simulink model "HPF"  (R2022a)
settings: Solver=VariableStepAuto  StartTime=0.0  StopTime=10.0  FixedStep=.000000001  RelTol=1e-3
values from neighbouring files (symbols this model uses):
  HPF_Sine_Amplitude = 1    [Run_Sim_HPF.m]
  HPF_Sine_Freq = 100    [Run_Sim_HPF.m]
  Vary_Sine_Feq = Start_Freq:step:End_Freq    [Run_Sim_HPF.m]
libraries: dspfdesign x7, dspsrcs4 x5
settings Model: Creator=chadw  LastModifiedBy=chadw

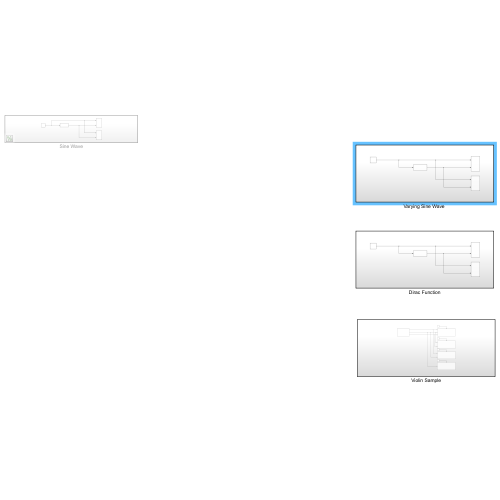
[thumbnail: Simulink's stored preview of the top-level diagram]
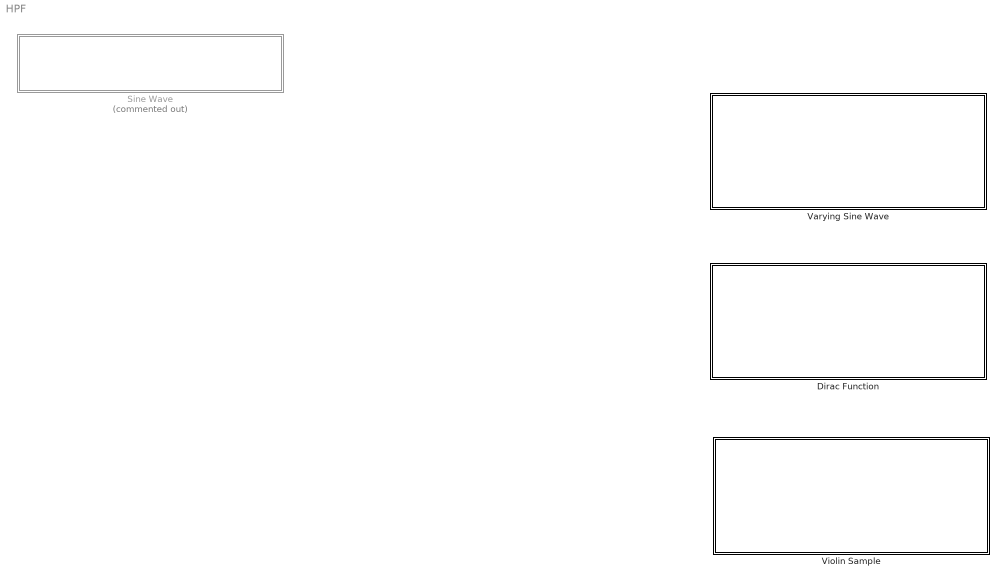
== system HPF ==
  Dirac Function : Subsystem
  Sine Wave : Subsystem  Commented=on
  "Varying Sine Wave " : Subsystem
  Violin Sample : Subsystem

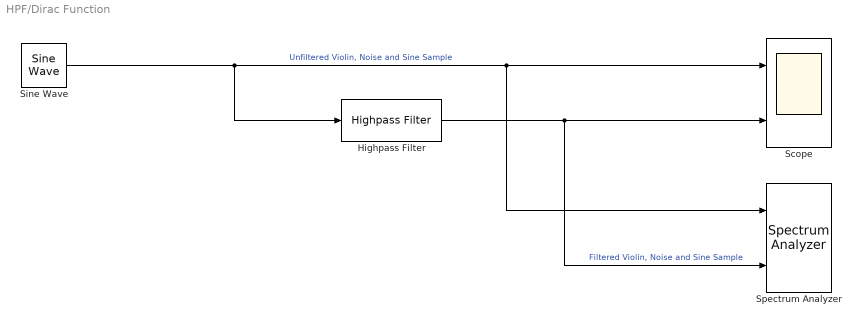
== system HPF/Dirac Function ==
  Highpass Filter : dspfdesign/Highpass Filter  FilterType=FIR  DesignForMinimumOrder=on  FilterOrder=50  StopbandFrequency=HPF_StopBand_Freq  PassbandFrequency=HPF_PassBand_Freq  StopbandAttenuation=HPF_StopBand_Amp  PassbandRipple=HPF_PassBand_Amp  InheritSampleRate=off  SampleRate=44100  SimulateUsing=Interpreted execution  roundingMode=Floor  coeffsDataTypeStr=fixdt(1,16)
  Scope : Scope  NumInputPorts=2
  Sine Wave : dspsrcs4/Sine Wave  Amplitude=1  Frequency=Vary_Sine_Feq  Phase=0  SampleMode=Discrete  OutComplex=Real  CompMethod=Trigonometric fcn  TableSize=Speed  SampleTime=1/1000  SamplesPerFrame=1  ResetState=Restart at time zero  OutputFrames=off  dataType=double  wordLen=16  udDataType=sfix(16)  fracBitsMode=Best precision  numFracBits=15  OutDataTypeStr=double  LastOutDataTypeStr=double
  Spectrum Analyzer : SpectrumAnalyzer  NumInputPorts=2
  wires:
  Sine Wave/1 -> Spectrum Analyzer/1, Scope/1, Highpass Filter/1  "Unfiltered Violin, Noise and Sine Sample"
  Highpass Filter/1 -> Spectrum Analyzer/2, Scope/2  "Filtered Violin, Noise and Sine Sample"

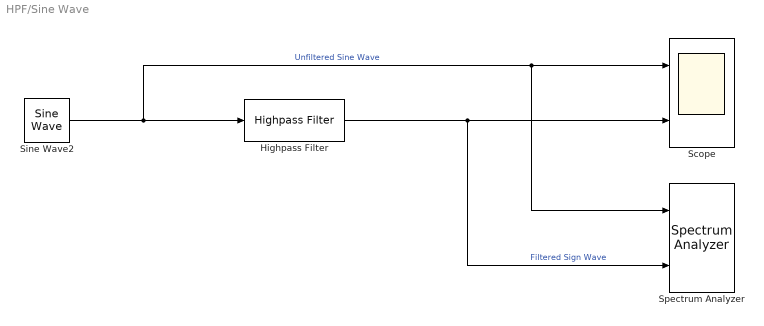
== system HPF/Sine Wave ==
  Highpass Filter : dspfdesign/Highpass Filter  FilterType=FIR  DesignForMinimumOrder=on  FilterOrder=50  StopbandFrequency=HPF_StopBand_Freq  PassbandFrequency=HPF_PassBand_Freq  StopbandAttenuation=HPF_StopBand_Amp  PassbandRipple=HPF_PassBand_Amp  InheritSampleRate=off  SampleRate=44100  SimulateUsing=Interpreted execution  roundingMode=Floor  coeffsDataTypeStr=fixdt(1,16)
  Scope : Scope  NumInputPorts=2
  Sine Wave2 : dspsrcs4/Sine Wave  Amplitude=HPF_Sine_Amplitude  Frequency=HPF_Sine_Freq  Phase=0  SampleMode=Discrete  OutComplex=Real  CompMethod=Trigonometric fcn  TableSize=Speed  SampleTime=1/1000  SamplesPerFrame=1  ResetState=Restart at time zero  OutputFrames=off  dataType=double  wordLen=16  udDataType=sfix(16)  fracBitsMode=Best precision  numFracBits=15  OutDataTypeStr=double  LastOutDataTypeStr=double
  Spectrum Analyzer : SpectrumAnalyzer  NumInputPorts=2
  wires:
  Sine Wave2/1 -> Scope/1, Spectrum Analyzer/1, Highpass Filter/1  "Unfiltered Sine Wave"
  Highpass Filter/1 -> Spectrum Analyzer/2, Scope/2  "Filtered Sign Wave"

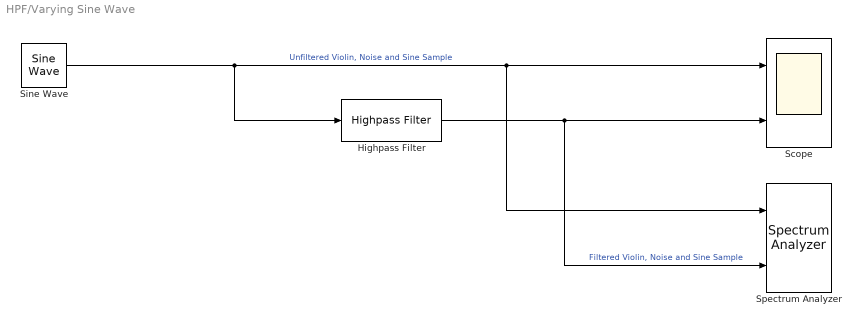
== system HPF/Varying Sine Wave  ==
  Highpass Filter : dspfdesign/Highpass Filter  FilterType=FIR  DesignForMinimumOrder=on  FilterOrder=50  StopbandFrequency=HPF_StopBand_Freq  PassbandFrequency=HPF_PassBand_Freq  StopbandAttenuation=HPF_StopBand_Amp  PassbandRipple=HPF_PassBand_Amp  InheritSampleRate=off  SampleRate=44100  SimulateUsing=Interpreted execution  roundingMode=Floor  coeffsDataTypeStr=fixdt(1,16)
  Scope : Scope  NumInputPorts=2
  Sine Wave : dspsrcs4/Sine Wave  Amplitude=1  Frequency=Vary_Sine_Feq  Phase=0  SampleMode=Discrete  OutComplex=Real  CompMethod=Trigonometric fcn  TableSize=Speed  SampleTime=1/1000  SamplesPerFrame=1  ResetState=Restart at time zero  OutputFrames=off  dataType=double  wordLen=16  udDataType=sfix(16)  fracBitsMode=Best precision  numFracBits=15  OutDataTypeStr=double  LastOutDataTypeStr=double
  Spectrum Analyzer : SpectrumAnalyzer  NumInputPorts=2
  wires:
  Highpass Filter/1 -> Scope/2, Spectrum Analyzer/2  "Filtered Violin, Noise and Sine Sample"
  Sine Wave/1 -> Highpass Filter/1, Scope/1, Spectrum Analyzer/1  "Unfiltered Violin, Noise and Sine Sample"

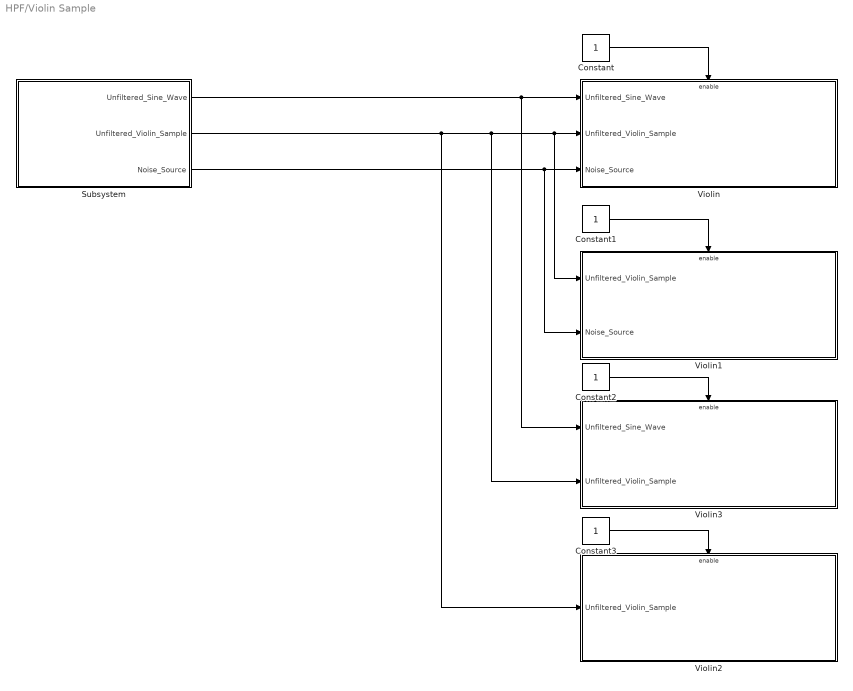
== system HPF/Violin Sample ==
  Constant{,1..3} (4 alike) : Constant  OutDataTypeStr=boolean
  Subsystem : Subsystem
  Violin : Subsystem
  Violin1 : Subsystem
  Violin2 : Subsystem
  Violin3 : Subsystem
  wires:
  Constant/1 -> Violin/Enable
  Subsystem/2(Unfiltered_Violin_Sample) -> Violin2/1(Unfiltered_Violin_Sample), Violin3/2(Unfiltered_Violin_Sample), Violin1/1(Unfiltered_Violin_Sample), Violin/2(Unfiltered_Violin_Sample)
  Constant3/1 -> Violin2/Enable
  Subsystem/1(Unfiltered_Sine_Wave) -> Violin3/1(Unfiltered_Sine_Wave), Violin/1(Unfiltered_Sine_Wave)
  Subsystem/3(Noise_Source) -> Violin1/2(Noise_Source), Violin/3(Noise_Source)
  Constant1/1 -> Violin1/Enable
  Constant2/1 -> Violin3/Enable

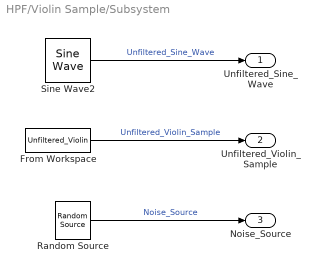
== system HPF/Violin Sample/Subsystem ==
  From Workspace : FromWorkspace  VariableName=Unfiltered_Violin  SampleTime=-1
  Random Source : dspsrcs4/Random Source  SrcType=Uniform  NormMethod=Ziggurat  CltLength=12  MinVal=0  MaxVal=1  MeanVal=0  VarVal=1  RepMode=Not repeatable  rawSeed=1  IsInherit=off  SampMode=Discrete  SampTime=1  SampFrame=1  DataType=Double  OutComplex=Real  OutputFrames=off
  Sine Wave2 : dspsrcs4/Sine Wave  Amplitude=HPF_Sine_Amplitude  Frequency=HPF_Sine_Freq  Phase=0  SampleMode=Discrete  OutComplex=Real  CompMethod=Trigonometric fcn  TableSize=Speed  SampleTime=1/1000  SamplesPerFrame=1  ResetState=Restart at time zero  OutputFrames=off  dataType=double  wordLen=16  udDataType=sfix(16)  fracBitsMode=Best precision  numFracBits=15  OutDataTypeStr=double  LastOutDataTypeStr=double
  Unfiltered_Sine_Wave : Outport
  Unfiltered_Violin_Sample : Outport  Port=2
  Noise_Source : Outport  Port=3
  wires:
  Random Source/1 -> Noise_Source/1  "Noise_Source"
  Sine Wave2/1 -> Unfiltered_Sine_Wave/1  "Unfiltered_Sine_Wave"
  From Workspace/1 -> Unfiltered_Violin_Sample/1  "Unfiltered_Violin_Sample"

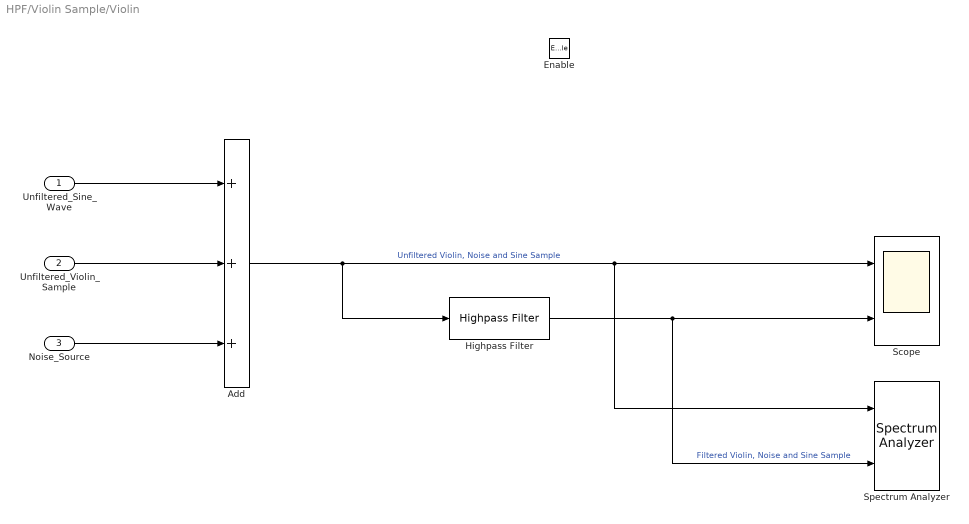
== system HPF/Violin Sample/Violin ==
  Unfiltered_Sine_Wave : Inport
  Unfiltered_Violin_Sample : Inport  Port=2
  Noise_Source : Inport  Port=3
  Enable : EnablePort
  Add : Sum  Inputs=3
  Highpass Filter : dspfdesign/Highpass Filter  FilterType=FIR  DesignForMinimumOrder=on  FilterOrder=50  StopbandFrequency=HPF_StopBand_Freq  PassbandFrequency=HPF_PassBand_Freq  StopbandAttenuation=HPF_StopBand_Amp  PassbandRipple=HPF_PassBand_Amp  InheritSampleRate=off  SampleRate=44100  SimulateUsing=Interpreted execution  roundingMode=Floor  coeffsDataTypeStr=fixdt(1,16)
  Scope : Scope  NumInputPorts=2
  Spectrum Analyzer : SpectrumAnalyzer  NumInputPorts=2
  wires:
  Highpass Filter/1 -> Scope/2, Spectrum Analyzer/2  "Filtered Violin, Noise and Sine Sample"
  Add/1 -> Highpass Filter/1, Scope/1, Spectrum Analyzer/1  "Unfiltered Violin, Noise and Sine Sample"
  Unfiltered_Sine_Wave/1 -> Add/1
  Unfiltered_Violin_Sample/1 -> Add/2
  Noise_Source/1 -> Add/3

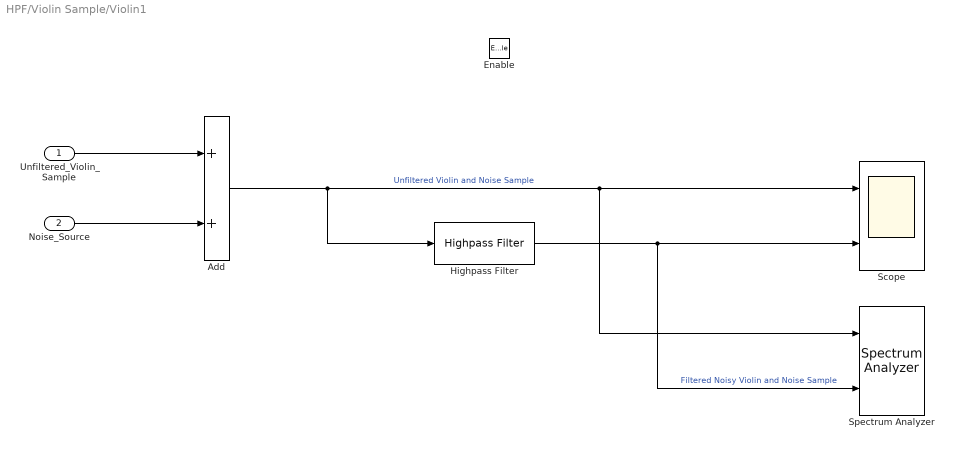
== system HPF/Violin Sample/Violin1 ==
  Unfiltered_Violin_Sample : Inport
  Noise_Source : Inport  Port=2
  Enable : EnablePort
  Add : Sum  Inputs=2
  Highpass Filter : dspfdesign/Highpass Filter  FilterType=FIR  DesignForMinimumOrder=on  FilterOrder=50  StopbandFrequency=HPF_StopBand_Freq  PassbandFrequency=HPF_PassBand_Freq  StopbandAttenuation=HPF_StopBand_Amp  PassbandRipple=HPF_PassBand_Amp  InheritSampleRate=off  SampleRate=44100  SimulateUsing=Interpreted execution  roundingMode=Floor  coeffsDataTypeStr=fixdt(1,16)
  Scope : Scope  NumInputPorts=2
  Spectrum Analyzer : SpectrumAnalyzer  NumInputPorts=2
  wires:
  Noise_Source/1 -> Add/2
  Add/1 -> Highpass Filter/1, Spectrum Analyzer/1, Scope/1  "Unfiltered Violin and Noise Sample"
  Highpass Filter/1 -> Spectrum Analyzer/2, Scope/2  "Filtered Noisy Violin and Noise Sample"
  Unfiltered_Violin_Sample/1 -> Add/1

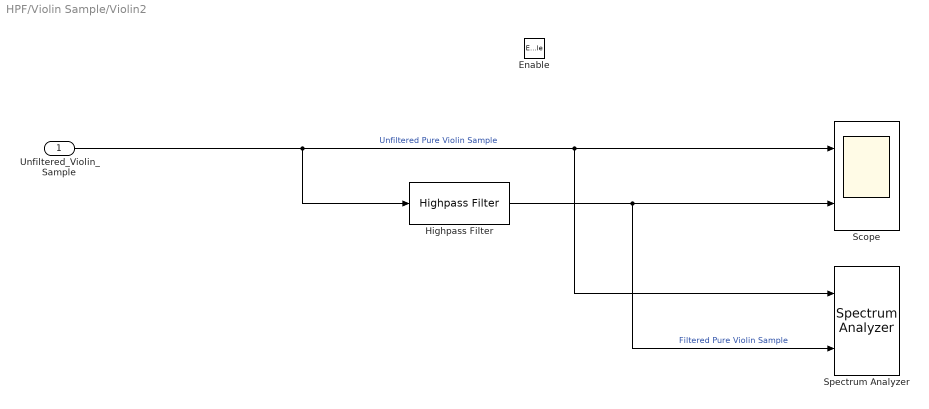
== system HPF/Violin Sample/Violin2 ==
  Unfiltered_Violin_Sample : Inport
  Enable : EnablePort
  Highpass Filter : dspfdesign/Highpass Filter  FilterType=FIR  DesignForMinimumOrder=on  FilterOrder=50  StopbandFrequency=HPF_StopBand_Freq  PassbandFrequency=HPF_PassBand_Freq  StopbandAttenuation=HPF_StopBand_Amp  PassbandRipple=HPF_PassBand_Amp  InheritSampleRate=off  SampleRate=44100  SimulateUsing=Interpreted execution  roundingMode=Floor  coeffsDataTypeStr=fixdt(1,16)
  Scope : Scope  NumInputPorts=2
  Spectrum Analyzer : SpectrumAnalyzer  NumInputPorts=2
  wires:
  Highpass Filter/1 -> Scope/2, Spectrum Analyzer/2  "Filtered Pure Violin Sample"
  Unfiltered_Violin_Sample/1 -> Scope/1, Spectrum Analyzer/1, Highpass Filter/1  "Unfiltered Pure Violin Sample"

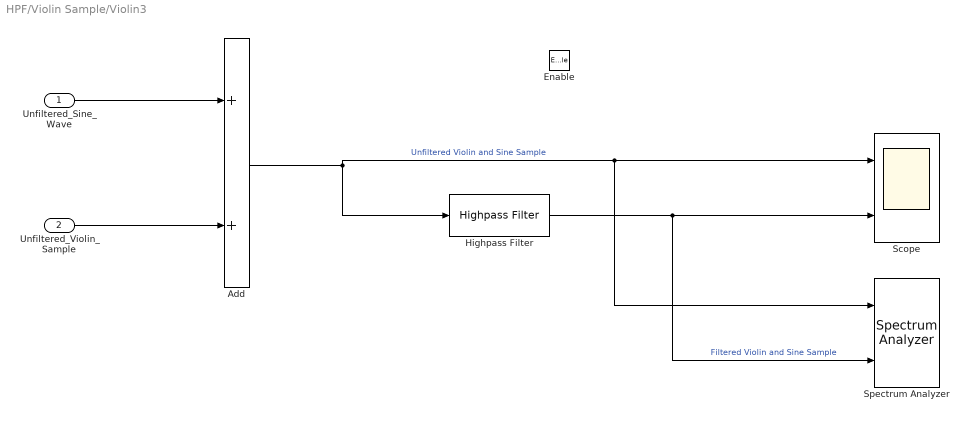
== system HPF/Violin Sample/Violin3 ==
  Unfiltered_Sine_Wave : Inport
  Unfiltered_Violin_Sample : Inport  Port=2
  Enable : EnablePort
  Add : Sum  Inputs=2
  Highpass Filter : dspfdesign/Highpass Filter  FilterType=FIR  DesignForMinimumOrder=on  FilterOrder=50  StopbandFrequency=HPF_StopBand_Freq  PassbandFrequency=HPF_PassBand_Freq  StopbandAttenuation=HPF_StopBand_Amp  PassbandRipple=HPF_PassBand_Amp  InheritSampleRate=off  SampleRate=44100  SimulateUsing=Interpreted execution  roundingMode=Floor  coeffsDataTypeStr=fixdt(1,16)
  Scope : Scope  NumInputPorts=2
  Spectrum Analyzer : SpectrumAnalyzer  NumInputPorts=2
  wires:
  Unfiltered_Violin_Sample/1 -> Add/2
  Unfiltered_Sine_Wave/1 -> Add/1
  Add/1 -> Spectrum Analyzer/1, Scope/1, Highpass Filter/1  "Unfiltered Violin and Sine Sample"
  Highpass Filter/1 -> Spectrum Analyzer/2, Scope/2  "Filtered Violin and Sine Sample"
